simulink model "Case2_CLF_CBF_QP_Controller"  (R2026a)
settings: Solver=VariableStepAuto  StopTime=30
PreLoadFcn:
  | % Define variants
  | VSS_PATH_CTRL_PURE_PURSUIT=Simulink.Variant('VSS_PATH_CTRL_MODE==1');
  | VSS_PATH_CTRL_REAR_WHEEL=Simulink.Variant('VSS_PATH_CTRL_MODE==2');
  | % Select default variant
  | VSS_PATH_CTRL_MODE =1;
  | 
  | 
  | % Longitudinal PID
  | LongitudinalPID.Kp = 20;
  | LongitudinalPID.Ki = 0;
  | LongitudinalPID.Kd = 0;
  | LongitudinalPID.N = 100;
  | LongitudinalPID.MaxAccel = 80;
  | LongitudinalPID.SampleTime = 0.01;
  | 
  | % Steering PID
  | SteeringPID.Kp = 60;
  | SteeringPID.Ki = 0;
  | SteeringPID.Kd = 5;
  | SteeringPID.N = 10;
  | SteeringPID.MaxSpeed =  10;
  | SteeringPID.MinSpeed = -10;
  | SteeringPID.SampleTime = 0.01;
  | 
  | 
  | 
  | setSMVehicleVisuParameters;
  | 
  | % Load planner commands
  | load('PlannerCmdTests.mat');
  | % Assign one for testing:
  | plannerCmd = plannerCmdFwd;
  | % plannerCmd  = plannerCmdFwdBwd;
  | 
  | % Bus structure definition
  | load('PlannerBusStruct.mat');
  | 
  | % Rear Wheel Controller Parameters
  | RW.k_e = 0.2;    % 0.1
  | RW.k_theta = 1;   % 0.75
  | RW.SampleTime =  0.1;
  | RW.GoalRadius = 0.3;
  | 
  | % Pure pursuit parameters
  | PP.DesiredLinearVel = 5;
  | PP.MaxAngularVel  = 10;
  | PP.LookaheadDist  = 1;
  | PP.Wheelbase = 4;
  | PP.GoalRadius = 0.1;
  | PP.SampleTime = 0.1;
  | PP.LongitudinalPID.Kp = 20;
  | PP.LongitudinalPID.Ki = 0;
  | PP.LongitudinalPID.Kd = 0;
  | PP.LongitudinalPID.N = 100;
  | PP.LongitudinalPID.MaxLongAccel =  80;
  | PP.LongitudinalPID.MinLongAccel = -80;
  | 
  | % Spline ref
  | splineRef = [ 0 0 0;[plannerCmd.PathMatrix(1:plannerCmd.PathLengths(1),1:2,1),0*ones(length(plannerCmd.PathMatrix(1:plannerCmd.PathLengths(1),1,1)),1)]];
values from neighbouring files (symbols this model uses):
  m = max(2, ceil(Lseg/ds))    [Trajectory.m]    (also in plot_nmpc_result.m = NaN)
  s = [0; cumsum(hypot(diff(xs),diff(ys)))]    [Trajectory.m]    (also in plot_parking_mpc.m = evalin('base',name); plot_result.m = out.(names{k}))
  trajMatrix = [tvec, xd, yd, thd, vd, wd]    [Trajectory.m]    (also in plot_parking_mpc.m = evalin('base','trajMatrix'); plot_result.m = evalin('base','trajMatrix'))
undefined symbols (not defined in the file or in its folder): DiscIntNeverNeededParam, smvv, X, Y, Z
libraries: sm_lib x527, sm_vehicle_slalom_lib x48, fl_lib x40, fl_ps_legacy_lib x28, nesl_utility x13
(part 15 of 15)

== system Case2_CLF_CBF_QP_Controller/Robot Bicycle Model/Visualizer/SM_Car_Visu/Vehicle7/Steering_Wheel/Logo/LStick3 ==
  Stick : sm_lib/Body Elements/Brick Solid  BrickDimensions=[smvv.steeringwheel.letterStick 0.001 0.001]  BrickDimensionsUnits=m  ExportEntireGeometry=off  InertiaType=PointMass  BasedOnType=Density  Density=1000  DensityUnits=kg/m^3  Mass=0.001  MassUnits=kg  CenterOfMass=[0 0 0]  CenterOfMassUnits=m  MomentsOfInertia=[1 1 1]  MomentsOfInertiaUnits=kg*m^2  ProductsOfInertia=[1 1 1]  ProductsOfInertiaUnits=kg*m^2  GraphicType=FromGeometry  MarkerShape=Sphere  MarkerSize=10  GraphicVisPropType=SimpleVisualProperties  GraphicDiffuseColor=smvv.steeringwheel.letterColor  GraphicOpacity=1.0  GraphicSpecularColor=[0.5 0.5 0.5 1.0]  GraphicAmbientColor=[0.15 0.15 0.15 1.0]  GraphicEmissiveColor=[0.0 0.0 0.0 1.0]  GraphicShininess=75  DoExposeReferenceFrame=on  SerializedFrames=<Frames/>
  X offset 1 : sm_lib/Frames and Transforms/Rigid Transform  RotationMethod=None  FollAlignAxisA=+X  BaseAlignAxisA=+Y  FollAlignAxisB=+Y  BaseAlignAxisB=+Z  RotationStandardAxis=+X  RotationAngle=0  RotationAngleUnits=deg  RotationArbitraryAxis=[0 0 1]  RotationSequenceAxes=FollowerAxes  RotationSequence=XYX  RotationSequenceAngles=[0 0 0]  RotationSequenceAnglesUnits=deg  RotationMatrix=[1 0 0; 0 1 0; 0 0 1]  Quaternion=[1 0 0 0]  TranslationMethod=StandardAxis  TranslationCartesianOffset=[0 0 0]  TranslationCartesianOffsetUnits=m  TranslationStandardAxis=-X  TranslationStandardOffset=0.5*smvv.steeringwheel.letterStick  TranslationStandardOffsetUnits=m  TranslationROffset=0  TranslationROffsetUnits=m  TranslationThetaOffset=0  TranslationThetaOffsetUnits=deg  TranslationZOffset=0  TranslationZOffsetUnits=m
  x offset 2 : sm_lib/Frames and Transforms/Rigid Transform  RotationMethod=None  FollAlignAxisA=+X  BaseAlignAxisA=+Y  FollAlignAxisB=+Y  BaseAlignAxisB=+Z  RotationStandardAxis=+X  RotationAngle=0  RotationAngleUnits=deg  RotationArbitraryAxis=[0 0 1]  RotationSequenceAxes=FollowerAxes  RotationSequence=XYX  RotationSequenceAngles=[0 0 0]  RotationSequenceAnglesUnits=deg  RotationMatrix=[1 0 0; 0 1 0; 0 0 1]  Quaternion=[1 0 0 0]  TranslationMethod=StandardAxis  TranslationCartesianOffset=[0 0 0]  TranslationCartesianOffsetUnits=m  TranslationStandardAxis=+X  TranslationStandardOffset=0.5*smvv.steeringwheel.letterStick  TranslationStandardOffsetUnits=m  TranslationROffset=0  TranslationROffsetUnits=m  TranslationThetaOffset=0  TranslationThetaOffsetUnits=deg  TranslationZOffset=0  TranslationZOffsetUnits=m
  Conn1 : PMIOPort  Side=Left
  Conn2 : PMIOPort  Port=2  Side=Right
  connections:
  X offset 1/RConn1 -- Conn1/RConn1
  x offset 2/RConn1 -- Conn2/RConn1
  x offset 2/LConn1 -- Stick/RConn1 -- X offset 1/LConn1

== system Case2_CLF_CBF_QP_Controller/Robot Bicycle Model/Visualizer/SM_Car_Visu/Vehicle7/Steering_Wheel/Logo/LStick4 ==
  Stick : sm_lib/Body Elements/Brick Solid  BrickDimensions=[smvv.steeringwheel.letterStick 0.001 0.001]  BrickDimensionsUnits=m  ExportEntireGeometry=off  InertiaType=PointMass  BasedOnType=Density  Density=1000  DensityUnits=kg/m^3  Mass=0.001  MassUnits=kg  CenterOfMass=[0 0 0]  CenterOfMassUnits=m  MomentsOfInertia=[1 1 1]  MomentsOfInertiaUnits=kg*m^2  ProductsOfInertia=[1 1 1]  ProductsOfInertiaUnits=kg*m^2  GraphicType=FromGeometry  MarkerShape=Sphere  MarkerSize=10  GraphicVisPropType=SimpleVisualProperties  GraphicDiffuseColor=smvv.steeringwheel.letterColor  GraphicOpacity=1.0  GraphicSpecularColor=[0.5 0.5 0.5 1.0]  GraphicAmbientColor=[0.15 0.15 0.15 1.0]  GraphicEmissiveColor=[0.0 0.0 0.0 1.0]  GraphicShininess=75  DoExposeReferenceFrame=on  SerializedFrames=<Frames/>
  X offset 1 : sm_lib/Frames and Transforms/Rigid Transform  RotationMethod=None  FollAlignAxisA=+X  BaseAlignAxisA=+Y  FollAlignAxisB=+Y  BaseAlignAxisB=+Z  RotationStandardAxis=+X  RotationAngle=0  RotationAngleUnits=deg  RotationArbitraryAxis=[0 0 1]  RotationSequenceAxes=FollowerAxes  RotationSequence=XYX  RotationSequenceAngles=[0 0 0]  RotationSequenceAnglesUnits=deg  RotationMatrix=[1 0 0; 0 1 0; 0 0 1]  Quaternion=[1 0 0 0]  TranslationMethod=StandardAxis  TranslationCartesianOffset=[0 0 0]  TranslationCartesianOffsetUnits=m  TranslationStandardAxis=-X  TranslationStandardOffset=0.5*smvv.steeringwheel.letterStick  TranslationStandardOffsetUnits=m  TranslationROffset=0  TranslationROffsetUnits=m  TranslationThetaOffset=0  TranslationThetaOffsetUnits=deg  TranslationZOffset=0  TranslationZOffsetUnits=m
  Conn1 : PMIOPort  Side=Left
  connections:
  Stick/RConn1 -- X offset 1/LConn1
  X offset 1/RConn1 -- Conn1/RConn1

== system Case2_CLF_CBF_QP_Controller/Robot Bicycle Model/Visualizer/SM_Car_Visu/Vehicle7/Steering_Wheel/Logo/LStick5 ==
  Stick : sm_lib/Body Elements/Brick Solid  BrickDimensions=[smvv.steeringwheel.letterStick 0.001 0.001]  BrickDimensionsUnits=m  ExportEntireGeometry=off  InertiaType=PointMass  BasedOnType=Density  Density=1000  DensityUnits=kg/m^3  Mass=0.001  MassUnits=kg  CenterOfMass=[0 0 0]  CenterOfMassUnits=m  MomentsOfInertia=[1 1 1]  MomentsOfInertiaUnits=kg*m^2  ProductsOfInertia=[1 1 1]  ProductsOfInertiaUnits=kg*m^2  GraphicType=FromGeometry  MarkerShape=Sphere  MarkerSize=10  GraphicVisPropType=SimpleVisualProperties  GraphicDiffuseColor=smvv.steeringwheel.letterColor  GraphicOpacity=1.0  GraphicSpecularColor=[0.5 0.5 0.5 1.0]  GraphicAmbientColor=[0.15 0.15 0.15 1.0]  GraphicEmissiveColor=[0.0 0.0 0.0 1.0]  GraphicShininess=75  DoExposeReferenceFrame=on  SerializedFrames=<Frames/>
  X offset 1 : sm_lib/Frames and Transforms/Rigid Transform  RotationMethod=None  FollAlignAxisA=+X  BaseAlignAxisA=+Y  FollAlignAxisB=+Y  BaseAlignAxisB=+Z  RotationStandardAxis=+X  RotationAngle=0  RotationAngleUnits=deg  RotationArbitraryAxis=[0 0 1]  RotationSequenceAxes=FollowerAxes  RotationSequence=XYX  RotationSequenceAngles=[0 0 0]  RotationSequenceAnglesUnits=deg  RotationMatrix=[1 0 0; 0 1 0; 0 0 1]  Quaternion=[1 0 0 0]  TranslationMethod=StandardAxis  TranslationCartesianOffset=[0 0 0]  TranslationCartesianOffsetUnits=m  TranslationStandardAxis=-X  TranslationStandardOffset=0.5*smvv.steeringwheel.letterStick  TranslationStandardOffsetUnits=m  TranslationROffset=0  TranslationROffsetUnits=m  TranslationThetaOffset=0  TranslationThetaOffsetUnits=deg  TranslationZOffset=0  TranslationZOffsetUnits=m
  x offset 2 : sm_lib/Frames and Transforms/Rigid Transform  RotationMethod=None  FollAlignAxisA=+X  BaseAlignAxisA=+Y  FollAlignAxisB=+Y  BaseAlignAxisB=+Z  RotationStandardAxis=+X  RotationAngle=0  RotationAngleUnits=deg  RotationArbitraryAxis=[0 0 1]  RotationSequenceAxes=FollowerAxes  RotationSequence=XYX  RotationSequenceAngles=[0 0 0]  RotationSequenceAnglesUnits=deg  RotationMatrix=[1 0 0; 0 1 0; 0 0 1]  Quaternion=[1 0 0 0]  TranslationMethod=StandardAxis  TranslationCartesianOffset=[0 0 0]  TranslationCartesianOffsetUnits=m  TranslationStandardAxis=+X  TranslationStandardOffset=0.5*smvv.steeringwheel.letterStick  TranslationStandardOffsetUnits=m  TranslationROffset=0  TranslationROffsetUnits=m  TranslationThetaOffset=0  TranslationThetaOffsetUnits=deg  TranslationZOffset=0  TranslationZOffsetUnits=m
  Conn1 : PMIOPort  Side=Left
  Conn2 : PMIOPort  Port=2  Side=Right
  connections:
  X offset 1/RConn1 -- Conn1/RConn1
  x offset 2/RConn1 -- Conn2/RConn1
  x offset 2/LConn1 -- Stick/RConn1 -- X offset 1/LConn1

== system Case2_CLF_CBF_QP_Controller/Robot Bicycle Model/Visualizer/SM_Car_Visu/Vehicle7/Steering_Wheel/Logo/LStick6 ==
  Stick : sm_lib/Body Elements/Brick Solid  BrickDimensions=[2*smvv.steeringwheel.letterStick 0.001 0.001]  BrickDimensionsUnits=m  ExportEntireGeometry=off  InertiaType=PointMass  BasedOnType=Density  Density=1000  DensityUnits=kg/m^3  Mass=0.001  MassUnits=kg  CenterOfMass=[0 0 0]  CenterOfMassUnits=m  MomentsOfInertia=[1 1 1]  MomentsOfInertiaUnits=kg*m^2  ProductsOfInertia=[1 1 1]  ProductsOfInertiaUnits=kg*m^2  GraphicType=FromGeometry  MarkerShape=Sphere  MarkerSize=10  GraphicVisPropType=SimpleVisualProperties  GraphicDiffuseColor=smvv.steeringwheel.letterColor  GraphicOpacity=1.0  GraphicSpecularColor=[0.5 0.5 0.5 1.0]  GraphicAmbientColor=[0.15 0.15 0.15 1.0]  GraphicEmissiveColor=[0.0 0.0 0.0 1.0]  GraphicShininess=75  DoExposeReferenceFrame=on  SerializedFrames=<Frames/>
  X offset 1 : sm_lib/Frames and Transforms/Rigid Transform  RotationMethod=None  FollAlignAxisA=+X  BaseAlignAxisA=+Y  FollAlignAxisB=+Y  BaseAlignAxisB=+Z  RotationStandardAxis=+X  RotationAngle=0  RotationAngleUnits=deg  RotationArbitraryAxis=[0 0 1]  RotationSequenceAxes=FollowerAxes  RotationSequence=XYX  RotationSequenceAngles=[0 0 0]  RotationSequenceAnglesUnits=deg  RotationMatrix=[1 0 0; 0 1 0; 0 0 1]  Quaternion=[1 0 0 0]  TranslationMethod=StandardAxis  TranslationCartesianOffset=[0 0 0]  TranslationCartesianOffsetUnits=m  TranslationStandardAxis=-X  TranslationStandardOffset=smvv.steeringwheel.letterStick  TranslationStandardOffsetUnits=m  TranslationROffset=0  TranslationROffsetUnits=m  TranslationThetaOffset=0  TranslationThetaOffsetUnits=deg  TranslationZOffset=0  TranslationZOffsetUnits=m
  x offset 2 : sm_lib/Frames and Transforms/Rigid Transform  RotationMethod=None  FollAlignAxisA=+X  BaseAlignAxisA=+Y  FollAlignAxisB=+Y  BaseAlignAxisB=+Z  RotationStandardAxis=+X  RotationAngle=0  RotationAngleUnits=deg  RotationArbitraryAxis=[0 0 1]  RotationSequenceAxes=FollowerAxes  RotationSequence=XYX  RotationSequenceAngles=[0 0 0]  RotationSequenceAnglesUnits=deg  RotationMatrix=[1 0 0; 0 1 0; 0 0 1]  Quaternion=[1 0 0 0]  TranslationMethod=StandardAxis  TranslationCartesianOffset=[0 0 0]  TranslationCartesianOffsetUnits=m  TranslationStandardAxis=+X  TranslationStandardOffset=smvv.steeringwheel.letterStick  TranslationStandardOffsetUnits=m  TranslationROffset=0  TranslationROffsetUnits=m  TranslationThetaOffset=0  TranslationThetaOffsetUnits=deg  TranslationZOffset=0  TranslationZOffsetUnits=m
  Conn1 : PMIOPort  Side=Left
  Conn2 : PMIOPort  Port=2  Side=Right
  connections:
  X offset 1/LConn1 -- Stick/RConn1 -- x offset 2/LConn1
  x offset 2/RConn1 -- Conn2/RConn1
  X offset 1/RConn1 -- Conn1/RConn1

== system Case2_CLF_CBF_QP_Controller/Robot Bicycle Model/Visualizer/SM_Car_Visu/Vehicle7/Steering_Wheel/Logo/LStick7 ==
  Stick : sm_lib/Body Elements/Brick Solid  BrickDimensions=[smvv.steeringwheel.letterStick 0.001 0.001]  BrickDimensionsUnits=m  ExportEntireGeometry=off  InertiaType=PointMass  BasedOnType=Density  Density=1000  DensityUnits=kg/m^3  Mass=0.001  MassUnits=kg  CenterOfMass=[0 0 0]  CenterOfMassUnits=m  MomentsOfInertia=[1 1 1]  MomentsOfInertiaUnits=kg*m^2  ProductsOfInertia=[1 1 1]  ProductsOfInertiaUnits=kg*m^2  GraphicType=FromGeometry  MarkerShape=Sphere  MarkerSize=10  GraphicVisPropType=SimpleVisualProperties  GraphicDiffuseColor=smvv.steeringwheel.letterColor  GraphicOpacity=1.0  GraphicSpecularColor=[0.5 0.5 0.5 1.0]  GraphicAmbientColor=[0.15 0.15 0.15 1.0]  GraphicEmissiveColor=[0.0 0.0 0.0 1.0]  GraphicShininess=75  DoExposeReferenceFrame=on  SerializedFrames=<Frames/>
  X offset 1 : sm_lib/Frames and Transforms/Rigid Transform  RotationMethod=None  FollAlignAxisA=+X  BaseAlignAxisA=+Y  FollAlignAxisB=+Y  BaseAlignAxisB=+Z  RotationStandardAxis=+X  RotationAngle=0  RotationAngleUnits=deg  RotationArbitraryAxis=[0 0 1]  RotationSequenceAxes=FollowerAxes  RotationSequence=XYX  RotationSequenceAngles=[0 0 0]  RotationSequenceAnglesUnits=deg  RotationMatrix=[1 0 0; 0 1 0; 0 0 1]  Quaternion=[1 0 0 0]  TranslationMethod=StandardAxis  TranslationCartesianOffset=[0 0 0]  TranslationCartesianOffsetUnits=m  TranslationStandardAxis=-X  TranslationStandardOffset=0.5*smvv.steeringwheel.letterStick  TranslationStandardOffsetUnits=m  TranslationROffset=0  TranslationROffsetUnits=m  TranslationThetaOffset=0  TranslationThetaOffsetUnits=deg  TranslationZOffset=0  TranslationZOffsetUnits=m
  Conn1 : PMIOPort  Side=Left
  connections:
  X offset 1/RConn1 -- Conn1/RConn1
  Stick/RConn1 -- X offset 1/LConn1

== matlab function Case2_CLF_CBF_QP_Controller/Close To Goal / Extract Goal ==
  data: Waypoints input; Goal output size=[2 1]
function Goal = extractGoal(Waypoints)
%#codegen
b = isnan(Waypoints);
[rows,~] = find(b);
ridx = setdiff(1:size(Waypoints,1), sort(rows));
Goal = [Waypoints(ridx(end), 1) Waypoints(ridx(end), 2)]';

== matlab function Case2_CLF_CBF_QP_Controller/MATLAB Function ==
  data: pose input; v output; trajectory input; delta output; V_out output; h_out output; h_obs_out output; t input; qp_status output; e_theta_out output; e_y_out output; e_x_out output; u_out output; slack1_out output; slack2_out output; slack3_out output; active1_out output; active2_out output; active3_out output
function [v, delta, V_out, h_out, h_obs_out, qp_status, e_theta_out, e_y_out, e_x_out, u_out, ...
          slack1_out, slack2_out, slack3_out, active1_out, active2_out, active3_out] = clf_cbf_qp_trajectory_controller(pose, trajectory, t)
% =========================================================================
% v14.0 -- FREEZING FIX + BRAKING CAPS + SINGLE FALLBACK (patch on v13.4).
%   (1) v_bar frozen at v_prev (rate-limited previous command), not v_des:
%       the one-step-lag / O(a_max*dt) certificate bound is now literally
%       true.
%   (2) [v14.1] Braking-distance caps tried and REMOVED -- they deadlock
%       pass-close manoeuvres (see note above the QP bounds).
%   (3) The v13.4 safety-only re-solve is retired: with the soft CLF row
%       (slack ceiling 1e6) the primary QP is infeasible iff the hard rows
%       are infeasible, so that re-solve could essentially never succeed.
%       One fallback remains: the rate-limited brake (u = 0).
%   (4) Optional NEARER_ONLY switch: during the swing, only the nearer
%       parked car's rows stay hard (default off).
%   qp_status:  >=0 primary QP solved (exitflag);  -3 brake fallback,
%               no certified safety this cycle;  -4 park-stall detector.
%               (-2 retired.)
% =========================================================================
% v13.4 -- SAFETY-RESPECTING INFEASIBILITY FALLBACK (patch on v13.1).
%   DIAGNOSED PROBLEM (from closed-loop run "v11"): h_obs went NEGATIVE
%   (-2.463 at t=25.71s, i.e. the two padded safety envelopes overlapped
%   by ~0.36m -- a genuine safety-margin violation, not a benign result)
%   during a run with 154 faulted QP solves (exitflag<=0). The OLD
%   fallback on infeasibility was:
%       v = 0; u0 = 0;                    % <-- ignores ALL 10 CBF/ECBF rows
%   This is not a certified-safe command -- it's just "stop and hope."
%   Every faulted solve was a cycle where the hard safety constraint this
%   whole architecture exists to guarantee was simply not enforced.
%
%   FIX (this revision): on infeasibility, before giving up, solve a
%   SECOND, much simpler QP: drop the CLF row and the slack column
%   entirely, keep all 10 CBF/ECBF rows exactly as hard constraints, and
%   minimize control effort (biases toward braking to a stop while still
%   respecting steering limits). This keeps the applied command inside
%   the CBF invariance argument even when the full tracking+CLF problem
%   has no solution. Only if THIS safety-only QP also fails does the
%   controller drop to a rate-limited hard brake (v ramped toward 0 at
%   exactly a_max_cmd, guaranteed rate-feasible by construction -- the
%   same last-resort pattern used in the MPC-CBF controller's fallback).
%
%   qp_status now distinguishes the three cases:
%       >=0  : primary tracking+CLF QP solved normally (exitflag)
%       -2   : safety-only fallback QP was used (primary QP infeasible)
%       -3   : total fallback -- even the safety-only QP failed; rate-
%              limited brake applied, no QP-certified safety this cycle
%       -4   : (unchanged) solved, but park-stall detector fired
%
%   NOTE: this patch does not, by itself, reduce WHY the primary QP goes
%   infeasible during the tight S-swing (the code's own senior-engineer
%   caution below still applies -- 8 steering-actuated rows sharing one
%   delta can genuinely over-constrain the problem there). It only
%   ensures that when that happens, the FALLBACK command is still safety-
%   respecting instead of blindly ignoring the barriers. If exitflag<=0
%   or qp_status<=-2 remains frequent, the next step is reducing the
%   over-constraint itself (e.g. only enforcing the nearer car's rows as
%   hard during the swing), not loosening r_veh/r_margin.
%
% ---------------------------------------------------------------------
% v13.1 -- UNIFIED KANAYAMA-STYLE CLF (replaces split sigma/e_x design) +
%          TIMED forward tracking (to x=60) + GLIDE/PARK reactive reverse.
%   The forward-tracking CLF now uses ONE Lyapunov function over ALL THREE
%   errors, V = 0.5*(e_x^2+e_y^2+e_theta^2), instead of e_x handled by a
%   separate proportional law and (e_y,e_theta) folded into a sigma. Its
%   derivative's reference-yaw-rate cross-terms cancel exactly, leaving a
%   CLF row affine in v (free, via e_x's own term) and u (v frozen at v_bar
%   only in u's coefficient, exactly as the CBF rows already do). A bonus:
%   no manual gear-direction flip is needed any more (the old s_dir), since
%   reversing correctly flips the u-coefficient's sign on its own.
%   Forward: pure time-indexed reference tracking (clock-driven), no waiting.
%   Reverse: the reactive boundary-gliding vector field + nonlinear pose
%            regulator + unjam bursts (ported from the proven v10.1 park logic)
%            take over once the car reaches x=60. This invents a collision-free
%            reverse reactively, so it needs no planned reverse reference and
%            robustly seats the car -- unlike path-following, which stalls if
%            the reference path clips an obstacle.
%   Keeps: 16-output signature, RD2 rear ECBF, split activation flags, the QP.
%
% New in v10.1: active1/2/3 now ENCODE which circle of each obstacle is
%   binding, without adding any Simulink ports:
%       0 = none, 1 = REAR only (ECBF), 2 = FRONT only (CBF), 3 = BOTH.
%   Decode downstream:  rear = mod(active,2) >= 1 ;  front = active >= 2.
%   slack1/2/3 stay as the worst-case (min over that obstacle's rows), so
%   the glide-arming trigger and the "how close to binding" plot are
%   unchanged. The trigger backstop still fires on ANY red activation.
%
% Change from v9.0 (per supervisor's recommendation to use RD2):
%   The rear-ego circles of the RED and PINK cars are physically
%   relative-degree 2 in the steering channel (their center (x,y) carries
%   no theta, so u does not appear until h-ddot). v9.0 enforced them as
%   one-pole CBFs in the SPEED channel (a_u = 0). v10.0 replaces those with
%   full TWO-POLE ECBFs, steering-actuated, using the SAME construction as
%   obstacle 3:
%       h-ddot + (g1+g2) h-dot + g1 g2 h  >= 0,   poles at (-g1_car, -g2_car).
%   FRONT-ego circles remain relative-degree 1 (u already in h-dot) -> plain
%   one-pole CBF. Obstacle 3 unchanged (rear ECBF + front CBF).
%
% Row map (11 rows, z = [v; u; s]):
%   1,2  RED  rear-ego  x {A,B} : RD2 ECBF (steering)   NEW
%   3,4  RED  front-ego x {A,B} : RD1 CBF  (steering)
%   5,6  PINK rear-ego  x {A,B} : RD2 ECBF (steering)   NEW
%   7,8  PINK front-ego x {A,B} : RD1 CBF  (steering)
%   9    OBS3 rear-ego          : RD2 ECBF (steering)
%   10   OBS3 front-ego         : RD1 CBF  (steering)
%   11   CLF (soft)
%
% CAUTION (senior-engineer note, read before trusting this): all eight car
% rows plus obs3 are now steering-actuated and share the single, rate-limited
% delta. Two consequences to watch:
%   (a) FEASIBILITY. During the tight S-swing this may over-constrain the QP
%       -> qp_status <= 0 (fail-safe stop). Keep the poles GENTLE (start at
%       -2.5, do NOT raise g1_car/g2_car to "hug harder") and watch exitflag.
%   (b) LOW-SPEED AUTHORITY. The steering coefficient L_gL_f h ~ v^2, so at
%       parking speed (v small) steering has weak authority over the rear
%       circles. If the rear rows go infeasible at low v, the belt-and-braces
%       fix is to ALSO keep a speed-channel row (see commented block below).
% =========================================================================

assert(numel(pose) == 3);
assert(size(trajectory,1) <= 2000);
assert(size(trajectory,2) == 6);
pose = pose(:).';

%% ---- Rate-limit bookkeeping (NEW in v6.11) ----
persistent v_prev lastT vdir_park parked_done slack_car_prev s_car_last t_arrive active1_prev
if isempty(v_prev)
    v_prev = 0;
    lastT  = t;
    vdir_park = 0;    % park reverse/forward direction latch (v7.1)
    parked_done = false;  % latched clean-stop flag (v7.3)
    slack_car_prev = 1e9; % previous step's worst car-CBF headroom (v8.0/v8.1)
    s_car_last     = 1e9; % ... and the step before that, for the rate estimate
    t_arrive       = -1;  % time the ego actually reached staging (v8.1)
    active1_prev   = 0;   % previous step's red-car activation flag (v8.2)
end
dt_step = max(t - lastT, 0);
lastT   = t;


CBF_ENABLE = true;


TRIG_MODE = 1;
s_trigger =  8.0;  % SHARED threshold: arms the glide AND latches park.

                  
t_ttb     = 2.0;   % mode 2: latch this many seconds before predicted binding.


% With CBF_ENABLE = false the glide is forced off regardless, since it now
% depends on the CBF.
GLIDE_NEEDS_CBF = true;

%% =================================================================

% ---- FIXED class-K rate for the relative-degree-1 CBF rows ----
% (Was an adaptive QP variable in [0.75, 6.25]; adaptivity removed in v9.0 --
%  gamma is now a plain constant. Used by the FRONT circles, all RD1.)
gamma_cbf = 2.5;

a_max_cmd = 3.0;   % hard ceiling on |dv/dt| for the COMMANDED speed [m/s^2]

%% ---- Fixed parameters (match the Robot Bicycle Model mask) ----
L           = 3;              % wheelbase [m]
delta_max   = 60*pi/180;      % steering saturation [rad]
u_max       = tan(delta_max);
v_lim       = 5.0;            % speed command bound [m/s]
k_e         = 1;              % lateral->heading coupling gain [1/m], RESTORED
                              % in v13.3 (needed by sigma, see below)
e_theta_max = 75*pi/180;      % heading-error bound [rad] (diagnostics only)

%% ---- CLF / CBF / cost tuning knobs (unchanged from v6.2) ----

c3      = 3.0;    % CLF convergence rate
k_x     = 0.6;    % longitudinal correction gain [1/s]
k_goal  = 0.6;    % final-settle creep gain [1/s]
v_creep = 0.5;    % final-settle creep speed limit [m/s]
w_v     = 1.0;    % speed-tracking weight
w_u     = 0.5;    % steering-effort weight (around feed-forward)
p_s     = 100.0;  % CLF slack penalty

%% ---- Parked cars: centers, now with REAL two-circle footprints ----

x_obs1 = 55.00; y_obs1 = 21.0;   % RED car  (ahead of bay)  -- was 56.00
x_obs2 = 40.00; y_obs2 = 21.0;   % PINK car (behind bay)    -- was 39.00
margin_base = 0.4;
k_v_margin  = 0.05;
v_park_nom  = 0.8;
r_margin    = margin_base + k_v_margin*v_park_nom;

r_veh = 1.6;          % per-circle radius, both ego and parked cars (derivation above)
car_half_spacing = 1.5;   % parked car's own front/rear circle offset from its center

r_pair = r_veh + r_veh + r_margin;   % combined safe center-to-center distance, ANY ego/car circle pair

% Each parked car's two FIXED circle centers (heading assumed 0, aligned with the lane)
x_c1r = x_obs1 - car_half_spacing;  y_c1r = y_obs1;   % red car,  circle A (toward bay)
x_c1f = x_obs1 + car_half_spacing;  y_c1f = y_obs1;   % red car,  circle B (away from bay)
x_c2r = x_obs2 - car_half_spacing;  y_c2r = y_obs2;   % pink car, circle A (away from bay)
x_c2f = x_obs2 + car_half_spacing;  y_c2f = y_obs2;   % pink car, circle B (toward bay)

% ---- Obstacle 3: unplanned, on the straight approach (unchanged from v6.7) ----
x_obs3 = 26.6;  y_obs3 = 17;  r_obs3 = 1.2;   % re-centered on the straight
                                                  
r_safe3 = r_obs3 + r_margin;
g1_3 = 2.0;  g2_3 = 2.0; 

% ---- Rear-CAR ECBF poles (NEW in v10.0) ----
g1_car = 2.0;  g2_car = 2.0;

x = pose(1); y = pose(2); theta = pose(3);

%% ---- How much of the (padded) trajectory table is "real" ----
Nrows = size(trajectory,1);
nReal = Nrows;
for k = Nrows:-1:2
    if trajectory(k,1) > trajectory(k-1,1) + 1e-9
        nReal = k;
        break;
    end
end
nReal = max(nReal, 2);

t_ref      = trajectory(1:nReal,1);
x_ref_tab  = trajectory(1:nReal,2);
y_ref_tab  = trajectory(1:nReal,3);
th_ref_tab = trajectory(1:nReal,4);
v_ref_tab  = trajectory(1:nReal,5);
k_ref_tab  = trajectory(1:nReal,6);

%% ---- Locate the forward->reverse GEAR CHANGE = the true staging row ----
nStage = nReal;
for k = 1:nReal
    if v_ref_tab(k) < -0.05
        nStage = max(k-1, 1);
        break;
    end
end
t_stage = t_ref(nStage);

%% ---- Reference lookup, CLAMPED to the staging row ----
tq = max(t_ref(1), min(t, t_stage));
x_ref0     = interp1(t_ref, x_ref_tab,  tq, 'linear');
y_ref0     = interp1(t_ref, y_ref_tab,  tq, 'linear');
theta_ref0 = interp1(t_ref, th_ref_tab, tq, 'linear');
v_ref0     = interp1(t_ref, v_ref_tab,  tq, 'linear');
kappa_ref0 = interp1(t_ref, k_ref_tab,  tq, 'linear');

%% ---- Synthesised "settle & hold at staging" ----
ref_moving_again = (t_arrive >= 0);
staging_hold = (t >= t_stage - 1e-9) && ~ref_moving_again;
if staging_hold
    v_ref0     = 0;
    kappa_ref0 = 0;
end

%% ---- Is there any FORWARD motion left in the approach? ----
rem_active = false;
if ~staging_hold
    for k = 1:nStage
        if t_ref(k) >= tq - 1e-9 && v_ref_tab(k) > 0.05
            rem_active = true;
            break;
        end
    end
end

%% ---- Park-phase goal pose (hardcoded, tied to the parked-car coords) --
x_goal     = (x_obs1 + x_obs2)/2 - L/2;   % 47.5 - 1.5 = 46.0 (body-centred)
y_goal     = y_obs1;                % curb line  = 21.0
theta_goal = 0;                     % park aligned with the lane

%% ---- Phase latch: approach -> park ----
x_stage = x_ref_tab(nStage);
y_stage = y_ref_tab(nStage);
persistent parkMode
if isempty(parkMode)
    parkMode = false;
end
dist_stage = hypot(x - x_stage, y - y_stage);

approach_done = ~rem_active && (t >= t_stage - 1e-9);
s_car_now     = slack_car_prev;                 % one-step-delayed, see below

%% ---- THE SHARED CBF TRIGGER (v8.2) ----
cbf_trigger = CBF_ENABLE && (x >= x_stage - 0.5);
s_car_last = s_car_now;

early_latch = approach_done && cbf_trigger;

if ~parkMode && early_latch
    parkMode = true;
end

%% ---- TWO-STAGE PARK: entry pose, then seat pose (NEW in v7.6) ----
R_des = 3.0;      % design radius of the seating S [m].
y_lane   = y_stage;
dy_park  = y_goal - y_lane;
c_phi    = 1 - dy_park/(2*R_des);
c_phi    = max(-1, min(1, c_phi));
phi_park = acos(c_phi);
x_entry  = x_goal + 2*R_des*sin(phi_park);

persistent parkStage
if isempty(parkStage)
    parkStage = 0;                        % 0 = GLIDE, 1 = SEAT
end
if parkMode && parkStage == 0 && x <= x_entry
    parkStage = 1;
end

%% ---- Stage 0 target: BOUNDARY-GLIDING VECTOR FIELD (NEW in v7.7) ----
h_on     = 14.0;
h_off    =  1.0;
r_follow =  3.8;

w_tan    =  2.0;
k_n      =  1.0;
Ld_glide =  3.5;
tau_gl   =  0.35;

persistent glide_dir
if isempty(glide_dir)
    glide_dir = [0, 0];
end

%% ---- Glide arming gate ----
persistent glide_armed
if isempty(glide_armed)
    glide_armed = false;
end
if ~CBF_ENABLE
    glide_armed = false;
elseif ~GLIDE_NEEDS_CBF
    glide_armed = true;           
elseif cbf_trigger
    glide_armed = true;
end
glide_on = CBF_ENABLE && glide_armed;

% ---- unjam burst state and constants (v7.8) ----
v_jam_thresh   = 0.10;
t_jam_confirm  = 0.40;
t_unjam        = 1.20;
v_unjam        = 0.80;
persistent jam_t unjam_t n_unjam
if isempty(jam_t)
    jam_t   = 0;
    unjam_t = 0;
    n_unjam = 0;
end

if parkStage == 0 && glide_on
    gvec = [x_goal - x, y_goal - y];
    gdir = gvec / max(hypot(gvec(1), gvec(2)), 1e-6);
    acc  = gdir;

    ox_all = [x_c1r, x_c1f, x_c2r, x_c2f];
    oy_all = [y_c1r, y_c1f, y_c2r, y_c2f];
    px_all = [x, x + L*cos(theta)];
    py_all = [y, y + L*sin(theta)];
    for io = 1:4
        for ip = 1:2
            Dxg = px_all(ip) - ox_all(io);
            Dyg = py_all(ip) - oy_all(io);
            dg  = hypot(Dxg, Dyg);
            hg  = dg^2 - r_pair^2;
            wg  = (h_on - hg) / (h_on - h_off);
            wg  = max(0, min(1, wg));
            if wg > 0
                ng = [Dxg, Dyg] / max(dg, 1e-6);
                tg = [-ng(2), ng(1)];
                if (tg(1)*gdir(1) + tg(2)*gdir(2)) < 0
                    tg = -tg;
                end
                acc = acc + wg*(w_tan*tg + k_n*(r_follow - dg)*ng);
            end
        end
    end
    dir_raw = acc / max(hypot(acc(1), acc(2)), 1e-6);

    if hypot(glide_dir(1), glide_dir(2)) < 1e-6
        glide_dir = dir_raw;
    else
        lam = min(1, dt_step/tau_gl);
        glide_dir = glide_dir + (dir_raw - glide_dir)*lam;
        glide_dir = glide_dir / max(hypot(glide_dir(1), glide_dir(2)), 1e-6);
    end

    x_tgt = x + Ld_glide*glide_dir(1);
    y_tgt = y + Ld_glide*glide_dir(2);
    theta_tgt = atan2(glide_dir(2), glide_dir(1)) + pi;
else
    glide_dir = [0, 0];
    x_tgt = x_goal;   y_tgt = y_goal;  theta_tgt = theta_goal;
end

%% ---- In park mode, replace the moving reference with the stage target ----
if parkMode
    x_ref0     = x_tgt;
    y_ref0     = y_tgt;
    theta_ref0 = theta_tgt;
    v_ref0     = 0;
    kappa_ref0 = 0;
end

%% ---- Tracking errors in the reference frame ----
err_vec     = [x - x_ref0, y - y_ref0];
tangent_ref = [cos(theta_ref0), sin(theta_ref0)];
normal_ref  = [-sin(theta_ref0), cos(theta_ref0)];
e_x = -(err_vec(1)*tangent_ref(1) + err_vec(2)*tangent_ref(2));
e_y =   err_vec(1)*normal_ref(1)  + err_vec(2)*normal_ref(2);
e_theta = mod((theta - theta_ref0) + pi, 2*pi) - pi;

%% ---- Gear-respecting desired speed & feed-forward steering ----
v_des = v_ref0 + k_x*e_x;
if v_ref0 > 0.05
    v_des = min(max(v_des, 0), v_lim);
elseif v_ref0 < -0.05
    v_des = max(min(v_des, 0), -v_lim);
else
    if rem_active
        v_des = 0;
    elseif abs(e_theta) < 0.3
        e_x_settled     = abs(e_x) < 0.03;
        e_theta_settled = abs(e_theta) < 0.02;
        if e_x_settled && e_theta_settled
            v_des = 0;
        elseif e_x_settled
            v_des = 0.15;
        else
            v_des = max(-v_creep, min(v_creep, k_goal*e_x));
        end
    else
        v_des = 0;
    end
end
%% ---- Park-mode pose regulator ----
park_uff  = 0;
clf_inert = false;
if parkMode
    k_rho_p    = 1.0;
    k_alpha_p  = 5.0;
    k_beta_p   = -2.5;
    v_park_max = 1.5;

    dx_g   = x_tgt - x;
    dy_g   = y_tgt - y;
    rho_g  = hypot(dx_g, dy_g);
    alpha0 = mod((atan2(dy_g, dx_g) - theta) + pi, 2*pi) - pi;
    
    if rho_g >= 0.35
        if vdir_park == 0
            if cos(alpha0) <= 0, vdir_park = -1; else, vdir_park = 1; end
        elseif vdir_park == -1 && cos(alpha0) >  0.4
            vdir_park = 1;
        elseif vdir_park ==  1 && cos(alpha0) < -0.4
            vdir_park = -1;
        end
    end
    if vdir_park == 0
        vdir_park = -1;
    end

    if vdir_park < 0
        alpha = mod((alpha0 - pi) + pi, 2*pi) - pi;
    else
        alpha = alpha0;
    end
    beta  = mod((theta_tgt - theta - alpha) + pi, 2*pi) - pi;

    v_mag = min(v_park_max, k_rho_p*rho_g);
    v_des = vdir_park * v_mag;

    omega   = k_alpha_p*alpha + k_beta_p*beta;
    
    v_den   = vdir_park * max(k_rho_p*rho_g, 0.25);
    park_uff = max(-u_max, min(u_max, L*omega / v_den));

    %% ---- UNJAM BURST ----
    if parkStage == 0
        if abs(v_prev) < v_jam_thresh
            jam_t = jam_t + dt_step;
        else
            jam_t = 0;
        end
        if jam_t > t_jam_confirm && unjam_t <= 0
            unjam_t = t_unjam;
            jam_t   = 0;
            n_unjam = n_unjam + 1;
        end
        if unjam_t > 0
            unjam_t   = unjam_t - dt_step;
            v_des     = v_unjam;
            vdir_park = 0;
        end
    else
        jam_t   = 0;
        unjam_t = 0;
    end
    
    if parkStage == 1 && (parked_done || (rho_g < 0.12 && abs(e_theta) < 0.035))
        parked_done = true;
        v_des    = 0;
        park_uff = 0;
    end

    clf_inert = true;
end

u_ff  = L*kappa_ref0;
u_ff  = max(-u_max, min(u_max, u_ff));
if parkMode
    u_ff = park_uff;
end
v_bar = v_prev;   % v14: freeze at the rate-limited PREVIOUS command, so the
               % certificate error is O(a_max_cmd*dt) -- the bound stated in
               % the dissertation Sec. 6.4. (v_des jumps by ~3 m/s at park
               % target switches; v_prev cannot.)

%% ---- Hybrid CLF: live e_x (unified) + proven sigma (e_y, e_theta) ----
omega_r = v_ref0 * kappa_ref0;
if v_bar >= 0
    s_dir = 1;
else
    s_dir = -1;
end
sigma = e_theta + s_dir*atan(k_e * e_y);
V     = 0.5*e_x^2 + 0.5*sigma^2;

%% ---- Ego circle centers ----
xr = x;              yr = y;
xf = x + L*cos(theta);  yf = y + L*sin(theta);

%% ---- RED car (obstacle 1): 2 ego circles x 2 car circles = 4 rows ----
Dx = xr - x_c1r; Dy = yr - y_c1r;
h_1rA  = Dx^2+Dy^2 - r_pair^2;
hd_1rA = 2*v_bar*(Dx*cos(theta)+Dy*sin(theta));
cu_1rA = 2*(v_bar^2/L)*(Dy*cos(theta)-Dx*sin(theta));
b_1rA  = 2*v_bar^2 + (g1_car+g2_car)*hd_1rA + g1_car*g2_car*h_1rA;
Dx = xr - x_c1f; Dy = yr - y_c1f;
h_1rB  = Dx^2+Dy^2 - r_pair^2;
hd_1rB = 2*v_bar*(Dx*cos(theta)+Dy*sin(theta));
cu_1rB = 2*(v_bar^2/L)*(Dy*cos(theta)-Dx*sin(theta));
b_1rB  = 2*v_bar^2 + (g1_car+g2_car)*hd_1rB + g1_car*g2_car*h_1rB;
Dx = xf - x_c1r; Dy = yf - y_c1r;
h_1fA = Dx^2+Dy^2 - r_pair^2;  a_1fA_v = 2*(Dx*cos(theta)+Dy*sin(theta));  a_1fA_u = 2*(Dy*cos(theta)-Dx*sin(theta))*v_bar;
Dx = xf - x_c1f; Dy = yf - y_c1f;
h_1fB = Dx^2+Dy^2 - r_pair^2;  a_1fB_v = 2*(Dx*cos(theta)+Dy*sin(theta));  a_1fB_u = 2*(Dy*cos(theta)-Dx*sin(theta))*v_bar;

%% ---- PINK car (obstacle 2): same pattern ----
Dx = xr - x_c2r; Dy = yr - y_c2r;
h_2rA  = Dx^2+Dy^2 - r_pair^2;
hd_2rA = 2*v_bar*(Dx*cos(theta)+Dy*sin(theta));
cu_2rA = 2*(v_bar^2/L)*(Dy*cos(theta)-Dx*sin(theta));
b_2rA  = 2*v_bar^2 + (g1_car+g2_car)*hd_2rA + g1_car*g2_car*h_2rA;
Dx = xr - x_c2f; Dy = yr - y_c2f;
h_2rB  = Dx^2+Dy^2 - r_pair^2;
hd_2rB = 2*v_bar*(Dx*cos(theta)+Dy*sin(theta));
cu_2rB = 2*(v_bar^2/L)*(Dy*cos(theta)-Dx*sin(theta));
b_2rB  = 2*v_bar^2 + (g1_car+g2_car)*hd_2rB + g1_car*g2_car*h_2rB;
Dx = xf - x_c2r; Dy = yf - y_c2r;
h_2fA = Dx^2+Dy^2 - r_pair^2;  a_2fA_v = 2*(Dx*cos(theta)+Dy*sin(theta));  a_2fA_u = 2*(Dy*cos(theta)-Dx*sin(theta))*v_bar;
Dx = xf - x_c2f; Dy = yf - y_c2f;
h_2fB = Dx^2+Dy^2 - r_pair^2;  a_2fB_v = 2*(Dx*cos(theta)+Dy*sin(theta));  a_2fB_u = 2*(Dy*cos(theta)-Dx*sin(theta))*v_bar;

%% ---- Obstacle 3, REAR-ego circle: HOCBF/ECBF, steering-actuated (RD2) ----
Dx3 = xr - x_obs3;  Dy3 = yr - y_obs3;
h_obs3 = Dx3^2 + Dy3^2 - r_safe3^2;
h3_dot = 2*v_bar*(Dx3*cos(theta) + Dy3*sin(theta));
c_u3   = 2*(v_bar^2/L)*(Dy3*cos(theta) - Dx3*sin(theta));
b_obs3 = 2*v_bar^2 + (g1_3+g2_3)*h3_dot + g1_3*g2_3*h_obs3;

%% ---- Obstacle 3, FRONT-ego circle: plain CBF, steering-actuated (RD1) ----
Dx3f = xf - x_obs3;  Dy3f = yf - y_obs3;
h_obs3f   = Dx3f^2 + Dy3f^2 - r_safe3^2;
a_obs3f_v = 2*(Dx3f*cos(theta) + Dy3f*sin(theta));
a_obs3f_u = 2*(Dy3f*cos(theta) - Dx3f*sin(theta))*v_bar;

%% ---- CLF row (soft) ----
den    = 1 + (k_e*e_y)^2;
clf_v  = -e_x;
clf_u  = sigma * (v_bar/L);
clf_c  = sigma * ( s_dir*k_e*v_bar*sin(e_theta)/den - omega_r ) ...
         + e_x*omega_r*e_y + e_x*v_ref0*cos(e_theta);
clf_V  = V;
if clf_inert
    clf_v = 0;
    clf_u = 0;
    clf_c = 0;
    clf_V = 0;
end

%% ---- Assemble the QP over z = [v; u; s] -- 11 rows total ----
H = 2*diag([w_v, w_u, p_s]);
f = [-2*w_v*v_des; -2*w_u*u_ff; 0];

A = [  0,          -cu_1rA,    0;    % row 1:  RED  rear-ego  x A  (RD2 ECBF)
       0,          -cu_1rB,    0;    % row 2:  RED  rear-ego  x B  (RD2 ECBF)
      -a_1fA_v,    -a_1fA_u,   0;    % row 3:  RED  front-ego x A  (RD1 CBF)
      -a_1fB_v,    -a_1fB_u,   0;    % row 4:  RED  front-ego x B  (RD1 CBF)
       0,          -cu_2rA,    0;    % row 5:  PINK rear-ego  x A  (RD2 ECBF)
       0,          -cu_2rB,    0;    % row 6:  PINK rear-ego  x B  (RD2 ECBF)
      -a_2fA_v,    -a_2fA_u,   0;    % row 7:  PINK front-ego x A  (RD1 CBF)
      -a_2fB_v,    -a_2fB_u,   0;    % row 8:  PINK front-ego x B  (RD1 CBF)
       0,          -c_u3,      0;    % row 9:  OBS3 rear-ego         (RD2 ECBF)
      -a_obs3f_v,  -a_obs3f_u, 0;    % row 10: OBS3 front-ego        (RD1 CBF)
       clf_v,       clf_u,    -1 ];  % row 11: CLF (soft, unified)
b = [ b_1rA; b_1rB; gamma_cbf*h_1fA; gamma_cbf*h_1fB; ...
      b_2rA; b_2rB; gamma_cbf*h_2fA; gamma_cbf*h_2fB; ...
      b_obs3; gamma_cbf*h_obs3f; ...
     -c3*clf_V - clf_c ];

if ~CBF_ENABLE
    A(1:10,:) = 0;
    b(1:10)   = 1e6;
end

%% ---- v14 OPTIONAL: only the NEARER car's rows stay hard during the swing ----
% (Relieves the S-swing over-constraint: 8 steering rows sharing one delta.
%  Default off. Set true if qp_status = -3 appears at stiff poles.)
NEARER_ONLY = false;
if NEARER_ONLY && parkMode
    if min([h_1rA,h_1rB,h_1fA,h_1fB]) < min([h_2rA,h_2rB,h_2fA,h_2fB])
        A(5:8,:) = 0;  b(5:8) = 1e6;   % PINK rows off this step
    else
        A(1:4,:) = 0;  b(1:4) = 1e6;   % RED rows off this step
    end
end

dv_max = a_max_cmd * max(dt_step, 1e-3);
v_lb = max(-v_lim, v_prev - dv_max);
v_ub = min( v_lim, v_prev + dv_max);

%% ---- v14.1 NOTE: an earlier revision inserted braking-distance caps on v
%%      here (v^2 <= 2*a_brake*gap as extra bounds). They were REMOVED: the
%%      stopping-envelope logic is correct for stop-for-obstacle missions
%%      but fences the car out of pass-close geometry -- it forced a crawl
%%      upstream of obstacle 3, and with v_bar = v_prev the steering
%%      coefficients (~v_bar^2/L) then collapsed, deadlocking the car in
%%      front of the obstacle. The proper speed-channel device for
%%      pass-close missions is a first-order CBF row in v (dissertation
%%      Sec. 9.2 future work), not a bound.
lb = [v_lb; -u_max; 0];
ub = [v_ub;  u_max; 1e6];

opts = optimoptions('quadprog', 'Display', 'off', 'Algorithm', 'active-set');
z0 = [ max(v_lb,  min(v_ub,  v_des)); ...
       max(-u_max, min(u_max, u_ff)); ...
       0 ];
[z, ~, exitflag, ~, lambda] = quadprog(H, f, A, b, [], [], lb, ub, z0, opts);

tol = 1e-4;
if exitflag > 0 && ~isempty(z)
    %% ---- PRIMARY QP solved normally ----
    v  = z(1);
    u0 = z(2);
    s_1rA = b(1)-A(1,:)*z;  s_1rB = b(2)-A(2,:)*z;  s_1fA = b(3)-A(3,:)*z;  s_1fB = b(4)-A(4,:)*z;
    s_2rA = b(5)-A(5,:)*z;  s_2rB = b(6)-A(6,:)*z;  s_2fA = b(7)-A(7,:)*z;  s_2fB = b(8)-A(8,:)*z;
    slack1 = min([s_1rA, s_1rB, s_1fA, s_1fB]);
    slack2 = min([s_2rA, s_2rB, s_2fA, s_2fB]);
    s_obs3r = b(9)  - A(9,:) *z;
    s_obs3f = b(10) - A(10,:)*z;
    slack3  = min(s_obs3r, s_obs3f);

    lam = lambda.ineqlin;
    a1_rear  = double( any(lam(1:2) > 0) || min(s_1rA,s_1rB) < tol );
    a1_front = double( any(lam(3:4) > 0) || min(s_1fA,s_1fB) < tol );
    a2_rear  = double( any(lam(5:6) > 0) || min(s_2rA,s_2rB) < tol );
    a2_front = double( any(lam(7:8) > 0) || min(s_2fA,s_2fB) < tol );
    a3_rear  = double( lam(9)  > 0 || s_obs3r < tol );
    a3_front = double( lam(10) > 0 || s_obs3f < tol );

    active1 = a1_rear + 2*a1_front;
    active2 = a2_rear + 2*a2_front;
    active3 = a3_rear + 2*a3_front;
    qp_status_raw = exitflag;
else
    %% ---- v14: SINGLE fallback -- rate-limited brake. The v13.4 safety-only
    %%      re-solve is retired: with the CLF row soft (slack ceiling 1e6),
    %%      the primary QP is infeasible IFF the hard rows are infeasible,
    %%      so that re-solve could essentially never succeed anyway. The
    %%      brake satisfies the rate constraint by construction. ----
    v  = sign(v_prev)*max(abs(v_prev) - dv_max, 0);
    u0 = 0;
    slack1 = NaN; slack2 = NaN; slack3 = NaN;
    active1 = 0;  active2 = 0;  active3 = 0;
    qp_status_raw = -3;      % total fallback: no QP-certified safety this cycle

end
delta = atan(u0);
v_prev = v;   % anchor next step's rate limit to what was ACTUALLY commanded

%% ---- Park-stall detector  ----
persistent stall_cnt
if isempty(stall_cnt)
    stall_cnt = 0;
end

park_stalled = false;
if parkMode && ~parked_done && abs(v) < 0.02
    stall_cnt = stall_cnt + 1;
else
    stall_cnt = 0;
end
if stall_cnt > round(1.5/max(dt_step,1e-3))    % motionless for ~1.5 s
    park_stalled = true;
end

%% ---- Diagnostics (original outputs unchanged) ----
V_out     = V;
h_out     = e_theta_max^2 - e_theta^2;
h_obs_out = min([h_1rA,h_1rB,h_1fA,h_1fB, h_2rA,h_2rB,h_2fA,h_2fB, h_obs3, h_obs3f]);
if park_stalled && qp_status_raw > 0
    qp_status = -4;          % solved, but deadlocked in park -- see note above
else
    qp_status = qp_status_raw;
end
e_theta_out = e_theta;
e_y_out     = e_y;
e_x_out     = e_x;
u_out       = u0;

slack1_out  = slack1;
slack2_out  = slack2;
slack3_out  = slack3;
active1_out = active1;
active2_out = active2;
active3_out = active3;
% ---- feed the glide arming latch ----
if CBF_ENABLE
    s_car = min(slack1, slack2);
    if ~isnan(s_car)
        slack_car_prev = s_car;
    end
    active1_prev = double(active1 > 0.5);
else
    slack_car_prev = 1e9;
    active1_prev   = 0;
end


end
% ================================

== matlab function Case2_CLF_CBF_QP_Controller/Robot Bicycle Model/wrapToPi ==
  data: qIn input; qOut output
function qOut = wrapToPi(qIn)
%#codegen

qOut = angdiff(0*qIn, qIn);
